simulink model "MJ1_2RC_EKF_v02_S1_PlantVerified"  (R2025b)
settings: Solver=FixedStepDiscrete  StartTime=0.0  StopTime=StopTime  FixedStep=1  RelTol=1e-3
undefined symbols (not defined in the file): C1_table, C2_table, OCV_table, Qref_Ah, R0_table, R1_table, R2_table, SOC0, SOC_bp, Ts, v1_0, v2_0
settings Model: Creator=louis  LastModifiedBy=louis

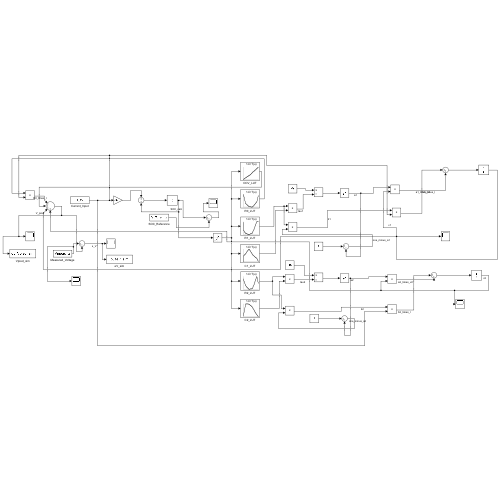
[thumbnail: Simulink's stored preview of the top-level diagram]
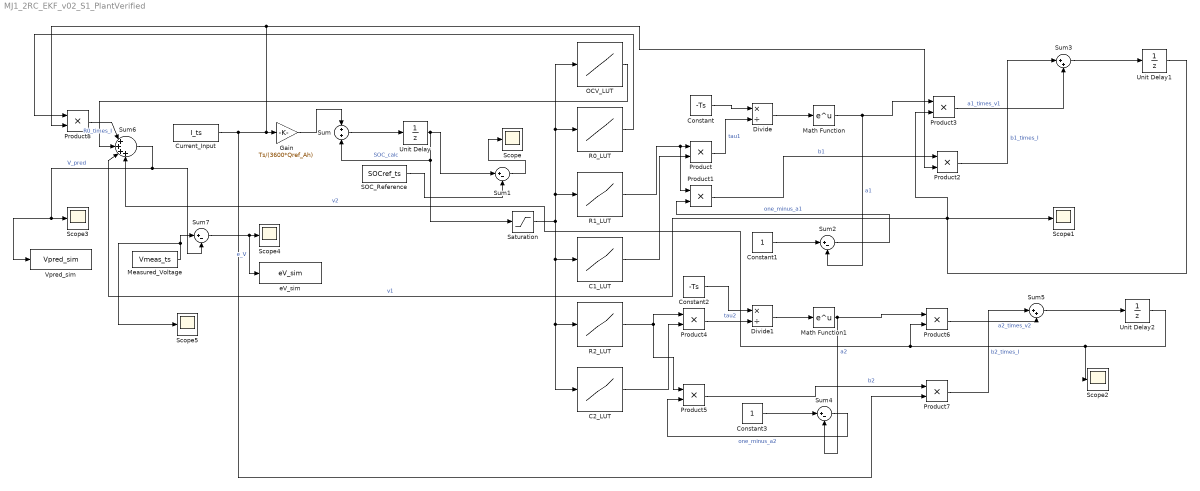
== system MJ1_2RC_EKF_v02_S1_PlantVerified ==
  C1_LUT : Lookup_n-D  NumberOfTableDimensions=1  BreakpointsForDimension1=SOC_bp  Table=C1_table  InternalRulePriority=Speed  RndMeth=Simplest
  C2_LUT : Lookup_n-D  NumberOfTableDimensions=1  BreakpointsForDimension1=SOC_bp  Table=C2_table  InternalRulePriority=Speed  RndMeth=Simplest
  Constant : Constant  Value=-Ts
  Constant1 : Constant
  Constant2 : Constant  Value=-Ts
  Constant3 : Constant
  Current_Input : FromWorkspace  VariableName=I_ts  SampleTime=1  Interpolate=off  OutputAfterFinalValue=Holding final value
  Divide : Product  Inputs=*/
  Divide1 : Product  Inputs=*/
  Gain : Gain  Gain=Ts/(3600*Qref_Ah)
  Math Function : Math
  Math Function1 : Math
  Measured_Voltage : FromWorkspace  VariableName=Vmeas_ts  SampleTime=1  Interpolate=off  OutputAfterFinalValue=Holding final value
  OCV_LUT : Lookup_n-D  NumberOfTableDimensions=1  BreakpointsForDimension1=SOC_bp  Table=OCV_table  InternalRulePriority=Speed  RndMeth=Simplest
  Product{,1..8} (9 alike) : Product
  R0_LUT : Lookup_n-D  NumberOfTableDimensions=1  BreakpointsForDimension1=SOC_bp  Table=R0_table  InternalRulePriority=Speed  RndMeth=Simplest
  R1_LUT : Lookup_n-D  NumberOfTableDimensions=1  BreakpointsForDimension1=SOC_bp  Table=R1_table  InternalRulePriority=Speed  RndMeth=Simplest
  R2_LUT : Lookup_n-D  NumberOfTableDimensions=1  BreakpointsForDimension1=SOC_bp  Table=R2_table  InternalRulePriority=Speed  RndMeth=Simplest
  SOC_Reference : FromWorkspace  VariableName=SOCref_ts  SampleTime=1  Interpolate=off  OutputAfterFinalValue=Holding final value
  Saturation : Saturate  UpperLimit=0.85  LowerLimit=0.17
  Scope{,1..5} (6 alike) : Scope
      Scope settings: ActiveDisplayYMinimum=-0.85672073625869916  ActiveDisplayYMaximum=0.7757637466107693
      Scope1 settings: ActiveDisplayYMinimum=-1  ActiveDisplayYMaximum=1
      Scope2 settings: ActiveDisplayYMinimum=-1  ActiveDisplayYMaximum=1  DataLoggingVariableName=ScopeData2
      Scope3 settings: DataLoggingVariableName=ScopeData3
      Scope4 settings: ActiveDisplayYMinimum=-1  ActiveDisplayYMaximum=1  DataLoggingVariableName=ScopeData4
      Scope5 settings: ActiveDisplayYMinimum=-1  ActiveDisplayYMaximum=1  DataLoggingVariableName=ScopeData5
  Sum : Sum
  Sum{1..2,4,7} (4 alike) : Sum  Inputs=|+-
  Sum3 : Sum  Inputs=|++
  Sum5 : Sum  Inputs=|++
  Sum6 : Sum  Inputs=|++++
  Unit Delay : UnitDelay  InitialCondition=SOC0  HasFrameUpgradeWarning=on
  Unit Delay1 : UnitDelay  InitialCondition=v1_0  HasFrameUpgradeWarning=on
  Unit Delay2 : UnitDelay  InitialCondition=v2_0  HasFrameUpgradeWarning=on
  Vpred_sim : ToWorkspace  VariableName=Vpred_sim  SaveFormat=Timeseries  SampleTime=-1
  eV_sim : ToWorkspace  VariableName=eV_sim  SaveFormat=Timeseries  SampleTime=-1
  wires:
  Current_Input/1 -> Product7/2, Product2/2, Product8/2, Gain/1
  Gain/1 -> Sum/1
  Sum/1 -> Unit Delay/1
  Unit Delay/1 -> Saturation/1, Sum/2, Sum1/1  "SOC_calc"
  SOC_Reference/1 -> Sum1/2
  Sum1/1 -> Scope/1
  Saturation/1 -> C2_LUT/1, R2_LUT/1, C1_LUT/1, R0_LUT/1, OCV_LUT/1, R1_LUT/1
  R1_LUT/1 -> Product1/1, Product/1
  C1_LUT/1 -> Product/2
  Constant/1 -> Divide/1
  Product/1 -> Divide/2  "tau1"
  Divide/1 -> Math Function/1
  Math Function/1 -> Product3/1, Sum2/2  "a1"
  Constant1/1 -> Sum2/1
  Sum2/1 -> Product1/2  "one_minus_a1"
  Product1/1 -> Product2/1  "b1"
  Unit Delay1/1 -> Product3/2, Scope1/1, Sum6/3  "v1"
  Product2/1 -> Sum3/1  "b1_times_I"
  Product3/1 -> Sum3/2  "a1_times_v1"
  Sum3/1 -> Unit Delay1/1
  R2_LUT/1 -> Product5/1, Product4/1
  C2_LUT/1 -> Product4/2
  Constant2/1 -> Divide1/1
  Product4/1 -> Divide1/2  "tau2"
  Divide1/1 -> Math Function1/1
  Sum4/1 -> Product5/2  "one_minus_a2"
  Product5/1 -> Product7/1  "b2"
  Math Function1/1 -> Sum4/2, Product6/1  "a2"
  Product6/1 -> Sum5/2  "a2_times_v2"
  Product7/1 -> Sum5/1  "b2_times_I"
  Sum5/1 -> Unit Delay2/1
  Constant3/1 -> Sum4/1
  Unit Delay2/1 -> Product6/2, Sum6/4, Scope2/1  "v2"
  R0_LUT/1 -> Product8/1
  Product8/1 -> Sum6/1  "R0_times_I"
  OCV_LUT/1 -> Sum6/2
  Sum6/1 -> Sum7/2, Vpred_sim/1, Scope3/1  "V_pred"
  Measured_Voltage/1 -> Sum7/1, Scope5/1
  Sum7/1 -> eV_sim/1, Scope4/1  "e_V"
